simulink model "ADMM_consensus"  (R2022b)
settings: Solver=FixedStepAuto  StartTime=0  StopTime=600*1001  FixedStep=200  RelTol=1e-3
values from neighbouring files (symbols this model uses):
  c = scaled_standard_constants    [Run_simulation.m]
settings Model: Creator=is123  LastModifiedBy=is123

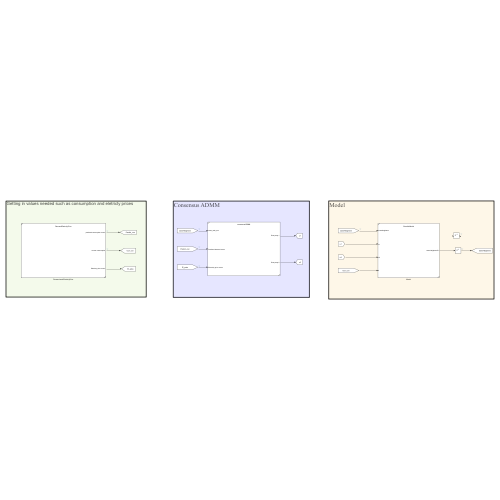
[thumbnail: Simulink's stored preview of the top-level diagram]
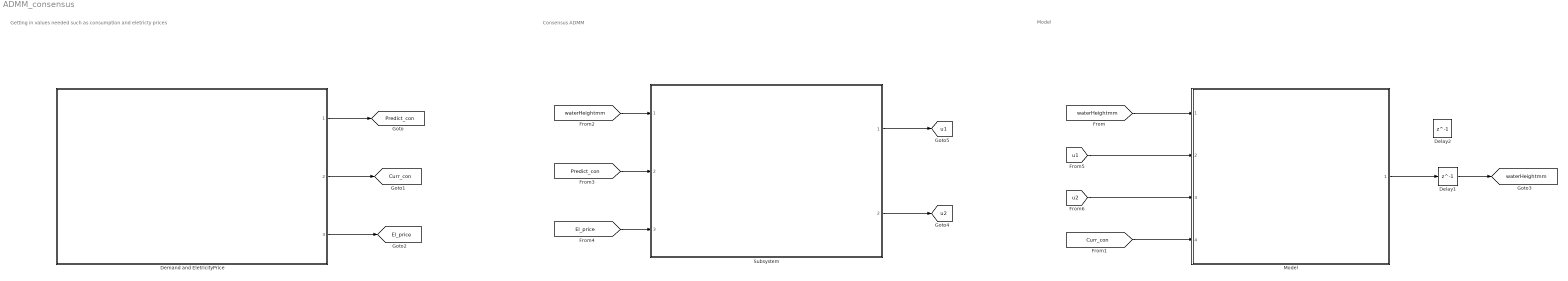
== system ADMM_consensus ==
  note: Getting in values needed such as consumption and eletricty prices
  note: Consensus ADMM
  note: Model
  Delay1 : Delay  DelayLength=1  InitialCondition=c.V/c.At*1e3
  Delay2 : Delay  DelayLength=1  InitialCondition=353
  Demand and EletricityPrice : Subsystem  ReferencedSubsystem=DemandEletricityPrice
  Model : Subsystem  ReferencedSubsystem=SimulinkModel
  Subsystem : Subsystem  ReferencedSubsystem=consensusADMM
  tag scope: Curr_con=global, El_price=global, Predict_con=global, u1=global, u2=global, waterHeightmm=global
  wires:
  Demand and EletricityPrice/1 -> [Predict_con]
  Demand and EletricityPrice/2 -> [Curr_con]
  Demand and EletricityPrice/3 -> [El_price]
  Model/1 -> Delay1/1
  Delay1/1 -> [waterHeightmm]
  [waterHeightmm] -> Model/1
  [Curr_con] -> Model/4
  [waterHeightmm] -> Subsystem/1
  [Predict_con] -> Subsystem/2
  [El_price] -> Subsystem/3
  Subsystem/2 -> [u2]
  Subsystem/1 -> [u1]
  [u1] -> Model/2
  [u2] -> Model/3
